simulink model "AM_DSB_SCBucle_RX_woRadio"  (R2024b)
settings: Solver=VariableStepAuto  StartTime=0.0  StopTime=inf  RelTol=1e-3
libraries: dspsrcs4 x4, dspfdesign x3, dspmlti4 x3, dspsnks4 x1, dspvision x1
settings Model: Creator=javier.alonsov  LastModifiedBy=javit

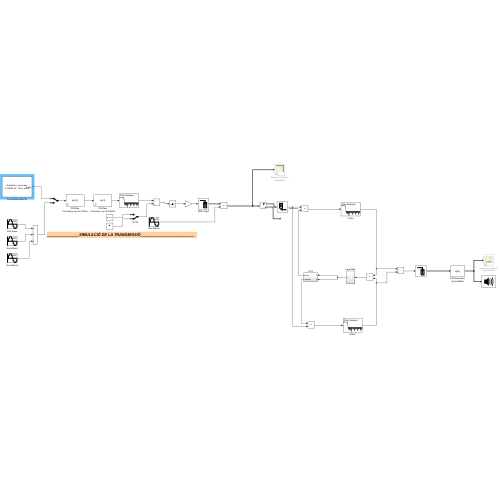
[thumbnail: Simulink's stored preview of the top-level diagram]
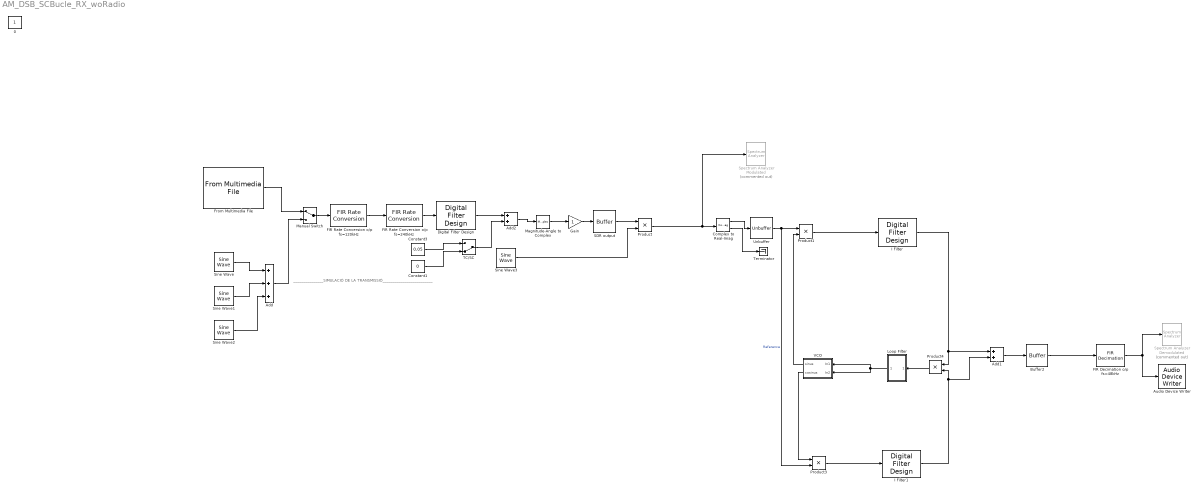
== system AM_DSB_SCBucle_RX_woRadio ==
  note: _______________SIMULACIÓ DE LA TRANSMISSIÓ_________________________
  Add : Sum  Inputs=+++
  Add1 : Sum
  Add2 : Sum
  Audio Device Writer : dspsnks4/Audio Device Writer  Driver=DirectSound  Device=Default  InheritSampleRate=on  SampleRate=44100  BitDepth=16-bit integer  BufferSize=4096  NumBuffers=10  DefaultOutputChannelMapping=on  OutputChannelMapping=1:2  OutputNumUnderrunSamples=off  DriverIdx=1  DeviceWarnFlag=''
  Buffer2 : Buffer  N=4096
  Complex to Real-Imag : ComplexToRealImag
  Constant1 : Constant  Value=0
  Constant3 : Constant  Value=0.05
  Digital Filter Design : dspfdesign/Digital Filter Design  mwdsp_browser_bugfix_var=off
  FIR Decimation o/p fs=48kHz : dspmlti4/FIR Decimation  FilterSource=Dialog parameters  h=firpm(200, [0 15e3 20e3 (240e3/2)]/(240e3/2), [1 1 0 0], [1 1], 20)  D=5  filtStruct=Direct form  FilterObject=Hm_firdecim  InputProcessing=Columns as channels (frame based)  framing=Allow multirate processing  AllowArbitraryInputLength=off  inputOffset=0  outputBufInitCond=0  roundingMode=Floor  overflowMode=off  firstCoeffDataTypeStr=Inherit: Same word length as input  firstCoeffMin=[]  firstCoeffMax=[]  firstCoeffLastDataTypeStr=Inherit: Same word length as input  outputDataTypeStr=Inherit: Same as accumulator  outputMin=[]  outputMax=[]  outputLastDataTypeStr=Inherit: Same as accumulator
  FIR Rate Conversion o/p fs=120kHz : dspmlti4/FIR Rate Conversion  FilterSource=Dialog parameters  L=5  h=firpm(50,[0 15e3 24e3 240e3/2]/(240e3/2),[1 1 0 0], [1 1],20)  M=2  FilterObject=FRC  rateMode=Enforce single-rate processing  AllowArbitraryInputLength=off  roundingMode=Floor  overflowMode=off  firstCoeffDataTypeStr=Inherit: Same word length as input  firstCoeffMin=[]  firstCoeffMax=[]  firstCoeffLastDataTypeStr=Inherit: Same word length as input  outputDataTypeStr=Inherit: Same as accumulator  outputMin=[]  outputMax=[]  outputLastDataTypeStr=Inherit: Same as accumulator
  FIR Rate Conversion o/p fs=240kHz : dspmlti4/FIR Rate Conversion  FilterSource=Auto  L=2  h=firpm(50,[0 15e3 30e3 600e3/2]/(600e3/2),[1 1 0 0], [1 1],20)  M=1  FilterObject=FRC  rateMode=Allow multirate processing  AllowArbitraryInputLength=off  roundingMode=Floor  overflowMode=off  firstCoeffDataTypeStr=Inherit: Same word length as input  firstCoeffMin=[]  firstCoeffMax=[]  firstCoeffLastDataTypeStr=Inherit: Same word length as input  outputDataTypeStr=Inherit: Same as accumulator  outputMin=[]  outputMax=[]  outputLastDataTypeStr=Inherit: Same as accumulator
  From Multimedia File : dspvision/From Multimedia File  inputFilename=C:\Users\javit\Documents\Curso25_26\Docencia\GET\SISCOM\LAB\SDR_3_DesmodAMNoCoherent\Grabacion_mono.wav  readRange=[1 Inf]  loop=on  numPlays=inf  outputStreams=Audio only  videoDataType=single  audioDataType=single  inheritSampleTime=on  userDefinedSampleTime=1/30  noAudioOutput=off  isIntensityVideo=off  fourcc=RGB  colorVideoFormat=One multidimensional signal  outputEOF=off  dataOrg=Column-major  audioFrameSize=600  computeAudioFrameSize=off  outSamplingMode=Sample based
      settings: LibrarySourceBlock=dspsrcs4/From Multimedia File
  Gain : Gain
  I Filter : dspfdesign/Digital Filter Design  mwdsp_browser_bugfix_var=off
  I Filter1 : dspfdesign/Digital Filter Design  mwdsp_browser_bugfix_var=off
  Loop Filter : Subsystem
  Magnitude-Angle to Complex : MagnitudeAngleToComplex  Input=Magnitude
  Manual Switch : ManualSwitch
  Product{,1,3..4} (4 alike) : Product
  SDR output : Buffer  N=4096
  Sine Wave : dspsrcs4/Sine Wave  Amplitude=0.05  Frequency=1e3  Phase=0  SampleMode=Discrete  OutComplex=Real  CompMethod=Trigonometric fcn  TableSize=Speed  SampleTime=1/48e3  SamplesPerFrame=600  ResetState=Restart at time zero  OutputFrames=off  dataType=double  wordLen=16  udDataType=sfix(16)  fracBitsMode=Best precision  numFracBits=15  OutDataTypeStr=double  LastOutDataTypeStr=double
  Sine Wave1 : dspsrcs4/Sine Wave  Amplitude=0.05  Frequency=5e3  Phase=0  SampleMode=Discrete  OutComplex=Real  CompMethod=Trigonometric fcn  TableSize=Speed  SampleTime=1/48e3  SamplesPerFrame=600  ResetState=Restart at time zero  OutputFrames=off  dataType=double  wordLen=16  udDataType=sfix(16)  fracBitsMode=Best precision  numFracBits=15  OutDataTypeStr=double  LastOutDataTypeStr=double
  Sine Wave2 : dspsrcs4/Sine Wave  Amplitude=0.05  Frequency=10e3  Phase=0  SampleMode=Discrete  OutComplex=Real  CompMethod=Trigonometric fcn  TableSize=Speed  SampleTime=1/48e3  SamplesPerFrame=600  ResetState=Restart at time zero  OutputFrames=off  dataType=double  wordLen=16  udDataType=sfix(16)  fracBitsMode=Best precision  numFracBits=15  OutDataTypeStr=double  LastOutDataTypeStr=double
  Sine Wave3 : dspsrcs4/Sine Wave  Amplitude=1  Frequency=39.85e3  Phase=0  SampleMode=Discrete  OutComplex=Complex  CompMethod=Trigonometric fcn  TableSize=Speed  SampleTime=1/240e3  SamplesPerFrame=4096  ResetState=Restart at time zero  OutputFrames=off  dataType=double  wordLen=16  udDataType=sfix(16)  fracBitsMode=Best precision  numFracBits=15  OutDataTypeStr=double  LastOutDataTypeStr=double
  Spectrum Analyzer Demodulated : SpectrumAnalyzer  Commented=on  WindowPosition=[1070.000000,603.000000,778.000000,224.000000,]  ScopeFrameLocation=window  Method=Welch  SampleRate=48000  AxesScaling=Manual  Span=240000  StartFrequency=-120000  StopFrequency=120000  AveragingMethod=Running  YLimits=[-180.94415229593105,48.14480110113395]  AllowFFTLengthLessThanSamplesPerUpdate=on  DefaultConfigurationName=spbscopes.SpectrumAnalyzerBlockCfg  IsFrequencyInputMode=0  FrequencyVectorPort=0  FrequencyVectorFromPort=0  FrequencyInputRBWPort=0  FrequencyInputRBWFromPort=0
  Spectrum Analyzer Modulated : SpectrumAnalyzer  Commented=on  WindowPosition=[1070.000000,261.000000,777.000000,407.000000,]  Visible=on  ScopeFrameLocation=window  Method=Welch  SampleRate=240000  AxesScaling=Manual  Span=240000  StartFrequency=-120000  StopFrequency=120000  AveragingMethod=Running  YLimits=[-146.72067730693476,43.804014640077718]  AllowFFTLengthLessThanSamplesPerUpdate=on  DefaultConfigurationName=spbscopes.SpectrumAnalyzerBlockCfg  IsFrequencyInputMode=0  FrequencyVectorPort=0  FrequencyVectorFromPort=0  FrequencyInputRBWPort=0  FrequencyInputRBWFromPort=0
  TC/SC : ManualSwitch  CurrentSetting=0
  Terminator : Terminator
  Unbuffer : Unbuffer
  VCO : Subsystem
  0 : Constant  IOType=siggen
  wires:
  FIR Rate Conversion o/p fs=120kHz/1 -> FIR Rate Conversion o/p fs=240kHz/1
  Manual Switch/1 -> FIR Rate Conversion o/p fs=120kHz/1
  From Multimedia File/1 -> Manual Switch/1
  Sine Wave/1 -> Add/1
  Sine Wave1/1 -> Add/2
  Sine Wave2/1 -> Add/3
  Add/1 -> Manual Switch/2
  FIR Rate Conversion o/p fs=240kHz/1 -> Digital Filter Design/1
  Digital Filter Design/1 -> Add2/1
  Magnitude-Angle to Complex/1 -> Gain/1
  Constant3/1 -> TC/SC/1
  TC/SC/1 -> Add2/2
  Constant1/1 -> TC/SC/2
  Gain/1 -> SDR output/1
  Add2/1 -> Magnitude-Angle to Complex/1
  SDR output/1 -> Product/1
  Sine Wave3/1 -> Product/2
  FIR Decimation o/p fs=48kHz/1 -> Audio Device Writer/1, Spectrum Analyzer Demodulated/1
  Unbuffer/1 -> Product3/2, Product1/1  "Reference"
  Complex to Real-Imag/2 -> Terminator/1
  Complex to Real-Imag/1 -> Unbuffer/1
  Product/1 -> Complex to Real-Imag/1, Spectrum Analyzer Modulated/1
  VCO/1(sinus) -> Product1/2
  VCO/2(cosinus) -> Product3/1
  Product1/1 -> I Filter/1
  Product3/1 -> I Filter1/1
  Loop Filter/1(Out1) -> VCO/2(In2), VCO/1(In1)
  Product4/1 -> Loop Filter/1(In1)
  I Filter/1 -> Product4/1, Add1/1
  I Filter1/1 -> Add1/2, Product4/2
  Buffer2/1 -> FIR Decimation o/p fs=48kHz/1
  Add1/1 -> Buffer2/1

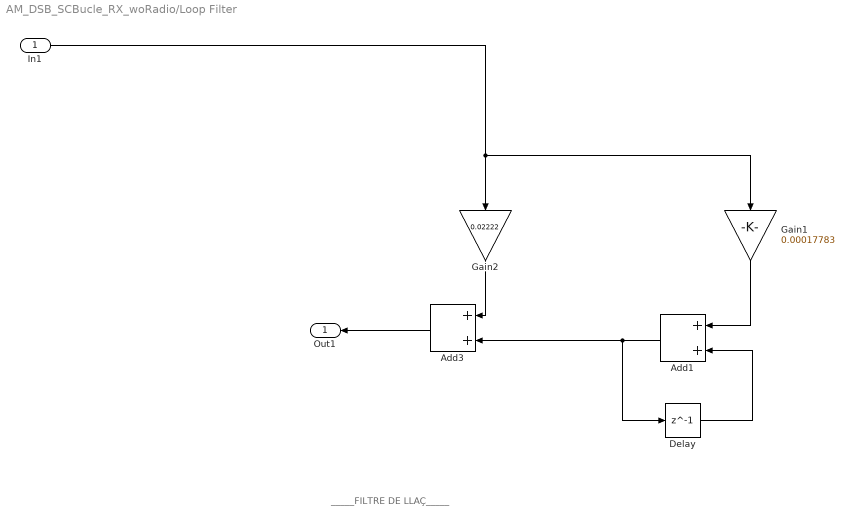
== system AM_DSB_SCBucle_RX_woRadio/Loop Filter ==
  note: _____FILTRE DE LLAÇ_____
  In1 : Inport
  Add1 : Sum
  Add3 : Sum  OutDataTypeStr=single  AccumDataTypeStr=single
  Delay : Delay  DelayLength=1  InitialCondition=0.00
  Gain1 : Gain  Gain=0.00017783  OutDataTypeStr=single
  Gain2 : Gain  Gain=0.02222  ParamDataTypeStr=single
  Out1 : Outport
  wires:
  Add1/1 -> Delay/1, Add3/2
  Add3/1 -> Out1/1
  In1/1 -> Gain2/1, Gain1/1
  Delay/1 -> Add1/2
  Gain2/1 -> Add3/1
  Gain1/1 -> Add1/1

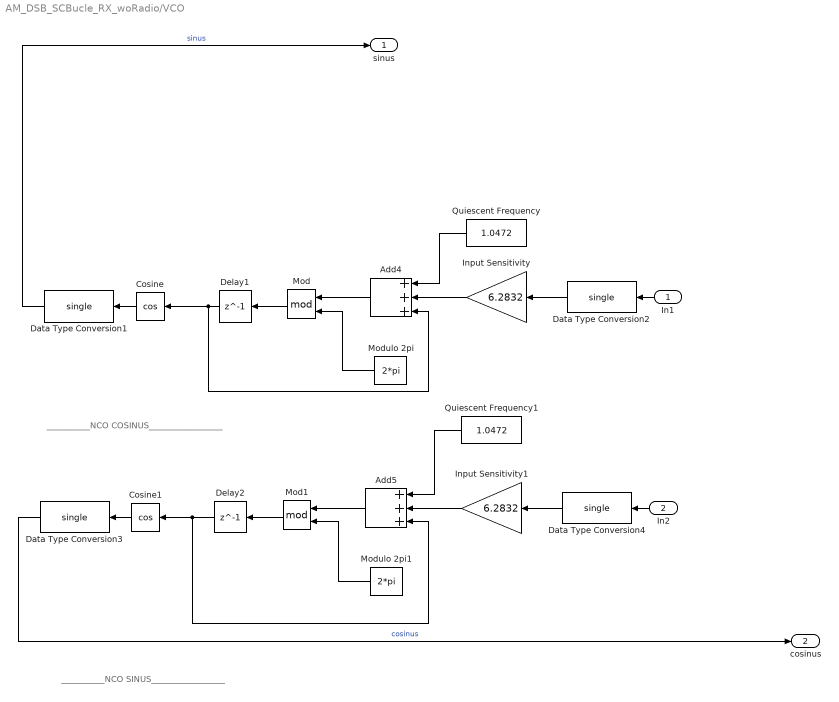
== system AM_DSB_SCBucle_RX_woRadio/VCO ==
  note: __________NCO COSINUS_________________
  note: __________NCO SINUS_________________
  In1 : Inport
  In2 : Inport  Port=2
  Add4 : Sum  Inputs=+++
  Add5 : Sum  Inputs=+++
  Cosine : Trigonometry  Operator=cos  OutputSignalType=real
  Cosine1 : Trigonometry  Operator=cos  OutputSignalType=real
  Data Type Conversion{1..4} (4 alike) : DataTypeConversion  OutDataTypeStr=single  SaturateOnIntegerOverflow=off  RndMeth=Floor
  Delay1 : Delay  DelayLength=1  InitialCondition=0
  Delay2 : Delay  DelayLength=1  InitialCondition=pi/2
  Input Sensitivity : Gain  Gain=6.2832
  Input Sensitivity1 : Gain  Gain=6.2832
  Mod : Math  Operator=mod
  Mod1 : Math  Operator=mod
  Modulo 2pi : Constant  Value=2*pi  SampleTime=1/240e3
  Modulo 2pi1 : Constant  Value=2*pi  SampleTime=1/240e3
  Quiescent Frequency : Constant  Value=1.0472  SampleTime=1/240e3
  Quiescent Frequency1 : Constant  Value=1.0472  SampleTime=1/240e3
  sinus : Outport
  cosinus : Outport  Port=2
  wires:
  Modulo 2pi1/1 -> Mod1/2
  Delay1/1 -> Cosine/1, Add4/3
  Cosine/1 -> Data Type Conversion1/1
  In1/1 -> Data Type Conversion2/1
  Data Type Conversion3/1 -> cosinus/1  "cosinus"
  Add5/1 -> Mod1/1
  Quiescent Frequency1/1 -> Add5/1
  Input Sensitivity1/1 -> Add5/2
  Input Sensitivity/1 -> Add4/2
  Mod1/1 -> Delay2/1
  Modulo 2pi/1 -> Mod/2
  Add4/1 -> Mod/1
  Quiescent Frequency/1 -> Add4/1
  Data Type Conversion2/1 -> Input Sensitivity/1
  Data Type Conversion4/1 -> Input Sensitivity1/1
  Data Type Conversion1/1 -> sinus/1  "sinus"
  Mod/1 -> Delay1/1
  In2/1 -> Data Type Conversion4/1
  Delay2/1 -> Cosine1/1, Add5/3
  Cosine1/1 -> Data Type Conversion3/1
